simulink model "dcm2"  (R2023a)
settings: Solver=ode45  StartTime=0.0  StopTime=2  RelTol=1e-3  EnableMultiTasking=on
InitFcn:
  | [dcm] = dcm2_init;
undefined symbols (not defined in the file or in its folder): dcm
settings Model: Creator=jkempkes  LastModifiedBy=herranz
settings SolverCC: AlgebraicLoopSolver=TrustRegion
settings DataIOCC: LimitDataPoints=on  SaveFormat=Array  SignalLoggingSaveFormat=ModelDataLogs  ReturnWorkspaceOutputs=off  SignalLoggingName=sigsOut
settings OptimizationCC: BooleanDataType=off  LifeSpan=inf
settings DebuggingCC: SaveWithParameterizedLinksMsg=none  UnderspecifiedInitializationDetection=Classic  MergeDetectMultiDrivingBlocksExec=none  SignalResolutionControl=TryResolveAllWithWarning  MultiTaskDSMMsg=warning  MultiTaskCondExecSysMsg=none  UnconnectedInputMsg=warning  UnconnectedOutputMsg=warning  UnconnectedLineMsg=warning  SFUnexpectedBacktrackingDiag=warning  SFNoUnconditionalDefaultTransitionDiag=warning  SFExecutionAtInitializationDiag=none  ArithmeticOperatorsInVariantConditions=warning
settings HardwareCC: ProdBitPerPointer=32  ProdBitPerSizeT=32  ProdBitPerPtrDiffT=32  ProdLargestAtomicFloat=None  ProdIntDivRoundTo=Undefined  ProdEndianess=Unspecified  ProdWordSize=32  ProdHWDeviceType=32-bit Generic  TargetUnknown=on
settings ModelReferenceCC: PropagateSignalLabelsOutOfModel=off
settings SFSimCC: SimUseLocalCustomCode=off  CustomCodeUndefinedFunction=UseInterfaceOnly
settings RTWCC: RTWUseLocalCustomCode=off
settings CodeAppCC: StateflowObjectComments=on
settings GRTTargetCC: TargetLangStandard=C89/C90 (ANSI)  CombineOutputUpdateFcns=off  GRTInterface=on
settings ConfigComp: CovMetricSettings=dw  CovSaveCumulativeToWorkspaceVar=on  CovSaveSingleToWorkspaceVar=on  CovExternalEMLEnable=off

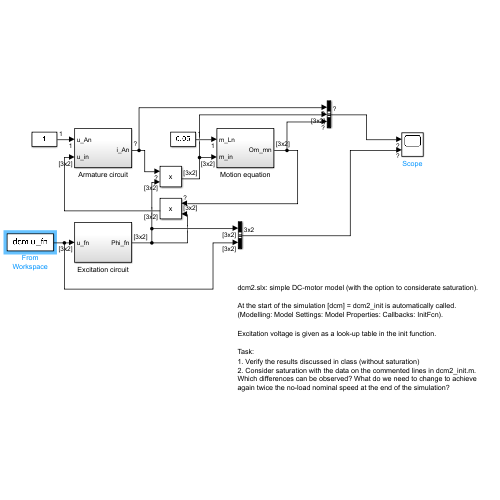
[thumbnail: Simulink's stored preview of the top-level diagram]
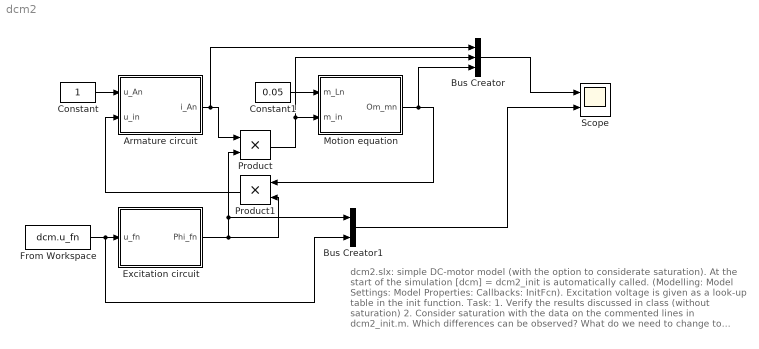
== system dcm2 ==
  note: dcm2.slx: simple DC-motor model (with the option to considerate saturation).
      |
      | At the start of the simulation [dcm] = dcm2_init is automatically called.
      | (Modelling: Model Settings: Model Properties: Callbacks: InitFcn).
      |
      | Excitation voltage is given as a look-up table in the init function.
      |
      | Task:
      | 1. Verify the results discussed in class (without saturation)
      | 2. Consider saturation with the data on the commented lines in dcm2_init.m. Which differences can be observed? What do we need to change to achieve again twice the no-load nominal speed at the end of the simulation?
  Armature circuit : Subsystem
  Bus Creator : BusCreator  Inputs=3
  Bus Creator1 : BusCreator  Inputs=2
  Constant : Constant
  Constant1 : Constant  Value=0.05
  Excitation circuit : Subsystem
  From Workspace : FromWorkspace  VariableName=dcm.u_fn  ZeroCross=off
  Motion equation : Subsystem
  Product : Product  InputSameDT=on  SaturateOnIntegerOverflow=on  OutDataTypeStr=Inherit: Same as first input
  Product1 : Product  InputSameDT=on  SaturateOnIntegerOverflow=on  OutDataTypeStr=Inherit: Same as first input
  Scope : Scope  NumInputPorts=2
  wires:
  Constant/1 -> Armature circuit/1(u_An)
  From Workspace/1 -> Bus Creator1/2, Excitation circuit/1(u_fn)
  Constant1/1 -> Motion equation/1(m_Ln)
  Motion equation/1(Om_mn) -> Bus Creator/3, Product1/1
  Armature circuit/1(i_An) -> Bus Creator/1, Product/1
  Excitation circuit/1(Phi_fn) -> Bus Creator1/1, Product/2, Product1/2
  Product1/1 -> Armature circuit/2(u_in)
  Product/1 -> Bus Creator/2, Motion equation/2(m_in)
  Bus Creator/1 -> Scope/1
  Bus Creator1/1 -> Scope/2

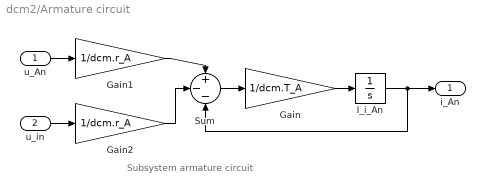
== system dcm2/Armature circuit ==
  note: Subsystem armature circuit
  u_An : Inport
  u_in : Inport  Port=2
  Gain : Gain  Gain=1/dcm.T_A  SaturateOnIntegerOverflow=on  OutDataTypeStr=Inherit: Same as input  ParamDataTypeStr=Inherit: Same as input
  Gain1 : Gain  Gain=1/dcm.r_A  SaturateOnIntegerOverflow=on  OutDataTypeStr=Inherit: Same as input  ParamDataTypeStr=Inherit: Same as input
  Gain2 : Gain  Gain=1/dcm.r_A  SaturateOnIntegerOverflow=on  OutDataTypeStr=Inherit: Same as input  ParamDataTypeStr=Inherit: Same as input
  I_i_An : Integrator
  Sum : Sum  Inputs=+--  InputSameDT=on  SaturateOnIntegerOverflow=on  OutDataTypeStr=Inherit: Same as first input
  i_An : Outport
  wires:
  Gain/1 -> I_i_An/1
  Sum/1 -> Gain/1
  u_An/1 -> Gain1/1
  u_in/1 -> Gain2/1
  Gain1/1 -> Sum/1
  Gain2/1 -> Sum/2
  I_i_An/1 -> Sum/3, i_An/1

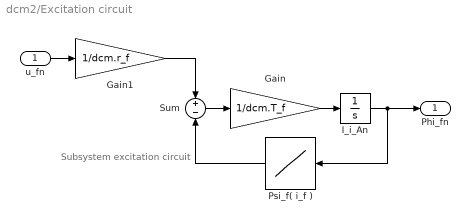
== system dcm2/Excitation circuit ==
  note: Subsystem excitation circuit
  u_fn : Inport
  Gain : Gain  Gain=1/dcm.T_f  SaturateOnIntegerOverflow=on  OutDataTypeStr=Inherit: Same as input  ParamDataTypeStr=Inherit: Same as input
  Gain1 : Gain  Gain=1/dcm.r_f  SaturateOnIntegerOverflow=on  OutDataTypeStr=Inherit: Same as input  ParamDataTypeStr=Inherit: Same as input
  I_i_An : Integrator  InitialCondition=dcm.Pfi_f0
  Psi_f( i_f ) : Lookup  InputValues=dcm.Phi_f  Table=dcm.i_f
  Sum : Sum  Inputs=+-  InputSameDT=on  SaturateOnIntegerOverflow=on  OutDataTypeStr=Inherit: Same as first input
  Phi_fn : Outport
  wires:
  u_fn/1 -> Gain1/1
  I_i_An/1 -> Psi_f( i_f )/1, Phi_fn/1
  Gain/1 -> I_i_An/1
  Sum/1 -> Gain/1
  Gain1/1 -> Sum/1
  Psi_f( i_f )/1 -> Sum/2

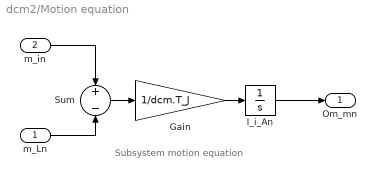
== system dcm2/Motion equation ==
  note: Subsystem motion equation
  m_Ln : Inport
  m_in : Inport  Port=2
  Gain : Gain  Gain=1/dcm.T_J  SaturateOnIntegerOverflow=on  OutDataTypeStr=Inherit: Same as input  ParamDataTypeStr=Inherit: Same as input
  I_i_An : Integrator  InitialCondition=dcm.Om_m0
  Sum : Sum  Inputs=+-  InputSameDT=on  SaturateOnIntegerOverflow=on  OutDataTypeStr=Inherit: Same as first input
  Om_mn : Outport
  wires:
  I_i_An/1 -> Om_mn/1
  Sum/1 -> Gain/1
  Gain/1 -> I_i_An/1
  m_in/1 -> Sum/1
  m_Ln/1 -> Sum/2
